simulink model "HalfAdder"  (R2016a)
settings: Solver=VariableStepAuto  StartTime=0.0  StopTime=10.0  RelTol=1e-3
settings Model: Creator=duyvu  LastModifiedBy=duyvu

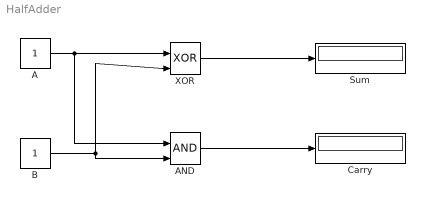
== system HalfAdder ==
  A : Constant
  AND : Logic  IconShape=distinctive  AllPortsSameDT=off  OutDataTypeStr=boolean
  B : Constant
  Carry : Display
  Sum : Display
  XOR : Logic  Operator=XOR  IconShape=distinctive  AllPortsSameDT=off  OutDataTypeStr=boolean
  wires:
  B/1 -> XOR/2, AND/2
  AND/1 -> Carry/1
  XOR/1 -> Sum/1
  A/1 -> AND/1, XOR/1
